simulink model "RA_Modes_Serial_HH"  (R2022b)
settings: Solver=FixedStepAuto  StartTime=0.0  StopTime=10.0  FixedStep=1e-3  RelTol=1e-3  EnableMultiTasking=on
undefined symbols (not defined in the file): A0, A1, D0, D1, D10, D11, D12, D13, D2, D3, D5, D6, D8, D9, PTA0, PTA1, PTA2, PTB2, PTB3, PTB9, PTC16, PTC17, PTC2, PTC4, PTD0, PTD1, PTD2, PTD3
libraries: etargetslib x22, frdmk64flib x20, dspstat3 x1
settings Model: ExtModeTrigDuration=5  Creator=haotianxue  LastModifiedBy=sarahalabdulrazzak
settings OptimizationCC: EnhancedBackFolding=on  PassReuseOutputArgsAs=Individual arguments  ZeroExternalMemoryAtStartup=off  ZeroInternalMemoryAtStartup=off  MaxStackSize=64  OptimizeBlockOrder=speed  DifferentSizesBufferReuse=on  OptimizationCustomize=off  EfficientTunableParamExpr=on
settings DebuggingCC: ParameterTunabilityLossMsg=error  UnconnectedInputMsg=warning  UnconnectedOutputMsg=warning  UnconnectedLineMsg=warning
settings HardwareCC: ProdBitPerPointer=32  ProdBitPerSizeT=32  ProdBitPerPtrDiffT=32  ProdLargestAtomicInteger=Long  ProdLargestAtomicFloat=Double  ProdWordSize=32  ProdHWDeviceType=ARM Compatible->ARM Cortex
settings ModelReferenceCC: EnableRefExpFcnMdlSchedulingChecks=on
settings SFSimCC: MATLABDynamicMemAlloc=off
settings RTWCC: Description=Embedded Coder  SystemTargetFile=ert.tlc  HardwareBoard=NXP FRDM-K64F  TLCOptions="-aInlineSetEventsForThisBaseRateFcn=TLC_FALSE -aSuppressMultiTaskScheduler=TLC_FALSE  -aRateBasedStepFcn=0"  TemplateMakefile=ert_default_tmf  Toolchain=GNU Tools for ARM Embedded Processors  DLArmComputeVersion=19.05
settings CodeAppCC: ForceParamTrailComments=on  IgnoreCustomStorageClasses=off  OperatorAnnotations=on  SimulinkDataObjDesc=on  SFDataObjDesc=on  InsertBlockDesc=on
settings ERTTargetCC: ExtModeTransport=4  ExtModeMexFile=sendToCommService

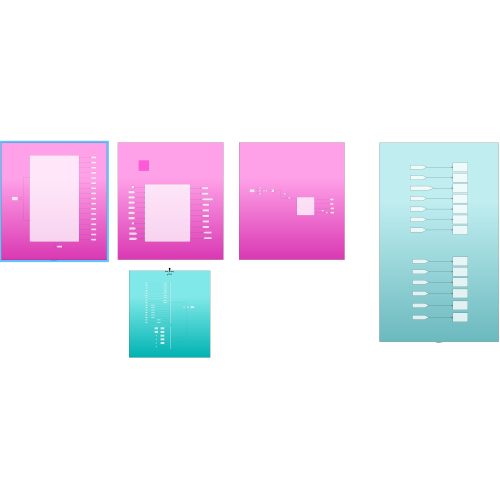
[thumbnail: Simulink's stored preview of the top-level diagram]
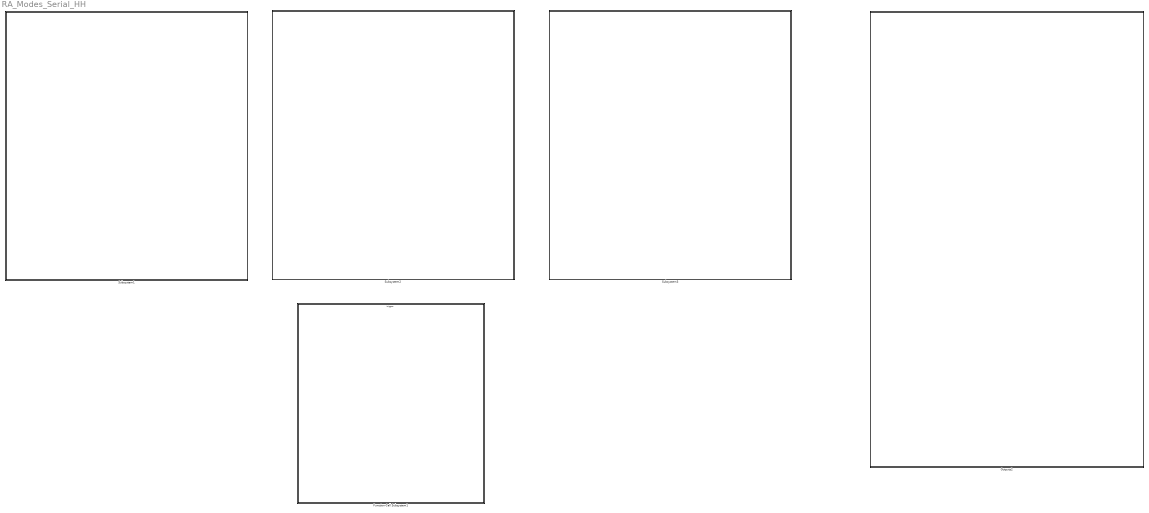
== system RA_Modes_Serial_HH ==
  Function-Call Subsystem1 : Subsystem  TreatAsAtomicUnit=on
  Outputs2 : Subsystem
  Subsystem1 : Subsystem
  Subsystem2 : Subsystem
  Subsystem3 : Subsystem

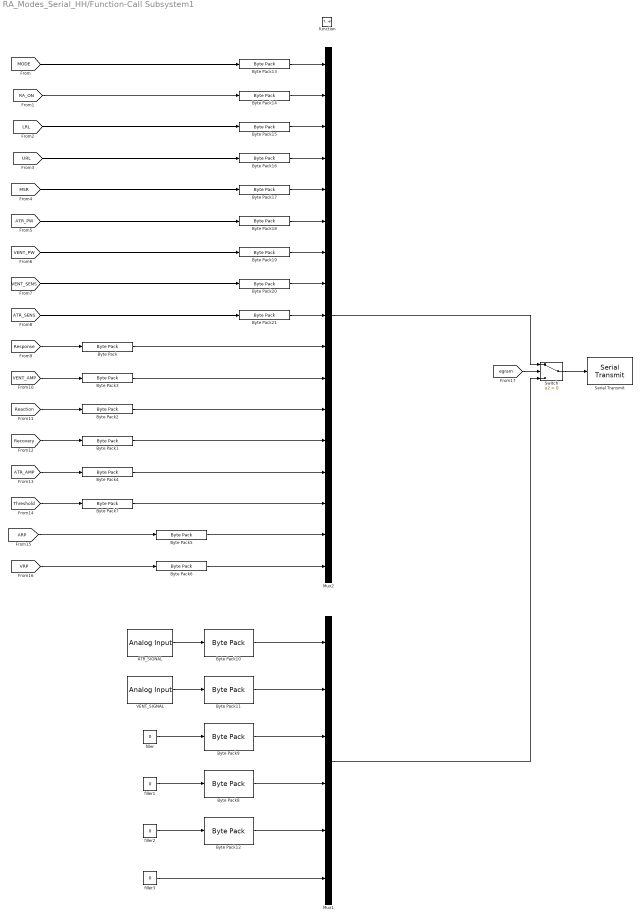
== system RA_Modes_Serial_HH/Function-Call Subsystem1 ==
  function : TriggerPort  TriggerType=function-call  IsSimulinkFunction=on  FunctionName=send_params  VariantControl=(inherit)
  ATR_SIGNAL : frdmk64flib/Analog Input  Whichpin=PTB2 (A0)  SampleTime=-1
  Byte Pack{,1..4,7,12} (7 alike) : etargetslib/Byte Pack  datatypes={'single'}  byteAlign=1
  Byte Pack{8..11} (4 alike) : etargetslib/Byte Pack  datatypes={'double'}  byteAlign=1
  Byte Pack{13..21} (9 alike) : etargetslib/Byte Pack  datatypes={'uint8'}  byteAlign=1
  Byte Pack5 : etargetslib/Byte Pack  datatypes={'uint16'}  byteAlign=1
  Byte Pack6 : etargetslib/Byte Pack  datatypes={'uint16'}  byteAlign=1
  Mux1 : Mux  Inputs=6
  Mux2 : Mux  Inputs=17
  Serial Transmit : frdmk64flib/Serial Transmit  SCIModule=0  Baudrate=uint32(9600)  Parity=None  StopBits=1  HardwareFlowControl=None  ByteOrder=LittleEndian  BlockingMode=on  OutputStatus=off
  Switch : Switch  Criteria=u2 > Threshold  SaturateOnIntegerOverflow=off  InputSameDT=off
  VENT_SIGNAL : frdmk64flib/Analog Input  Whichpin=PTB3 (A1)  SampleTime=-1
  filler : Constant  Value=0  OutDataTypeStr=double
  filler1 : Constant  Value=0  OutDataTypeStr=double
  filler2 : Constant  Value=0  OutDataTypeStr=single
  filler3 : Constant  Value=0  OutDataTypeStr=uint8
  wires:
  [VENT_SENS] -> Byte Pack20/1
  [ATR_SENS] -> Byte Pack21/1
  Byte Pack/1 -> Mux2/10
  Byte Pack1/1 -> Mux2/13
  Byte Pack2/1 -> Mux2/12
  Byte Pack3/1 -> Mux2/11
  Byte Pack4/1 -> Mux2/14
  Byte Pack5/1 -> Mux2/16
  Byte Pack6/1 -> Mux2/17
  [MODE] -> Byte Pack13/1
  [RA_ON] -> Byte Pack14/1
  [LRL] -> Byte Pack15/1
  [URL] -> Byte Pack16/1
  [MSR] -> Byte Pack17/1
  [ATR_PW] -> Byte Pack18/1
  [VENT_PW] -> Byte Pack19/1
  [Response] -> Byte Pack/1
  [VENT_AMP] -> Byte Pack3/1
  [Reaction] -> Byte Pack2/1
  [Recovery] -> Byte Pack1/1
  [ATR_AMP] -> Byte Pack4/1
  Byte Pack7/1 -> Mux2/15
  [Threshold] -> Byte Pack7/1
  [ARP] -> Byte Pack5/1
  [VRP] -> Byte Pack6/1
  Switch/1 -> Serial Transmit/1
  Mux2/1 -> Switch/1
  ATR_SIGNAL/1 -> Byte Pack10/1
  VENT_SIGNAL/1 -> Byte Pack11/1
  Mux1/1 -> Switch/3
  Byte Pack10/1 -> Mux1/1
  Byte Pack11/1 -> Mux1/2
  Byte Pack8/1 -> Mux1/4
  Byte Pack9/1 -> Mux1/3
  filler/1 -> Byte Pack9/1
  filler1/1 -> Byte Pack8/1
  Byte Pack12/1 -> Mux1/5
  filler2/1 -> Byte Pack12/1
  filler3/1 -> Mux1/6
  Byte Pack13/1 -> Mux2/1
  Byte Pack14/1 -> Mux2/2
  Byte Pack15/1 -> Mux2/3
  Byte Pack16/1 -> Mux2/4
  Byte Pack17/1 -> Mux2/5
  Byte Pack18/1 -> Mux2/6
  Byte Pack19/1 -> Mux2/7
  Byte Pack20/1 -> Mux2/8
  Byte Pack21/1 -> Mux2/9
  [egram] -> Switch/2

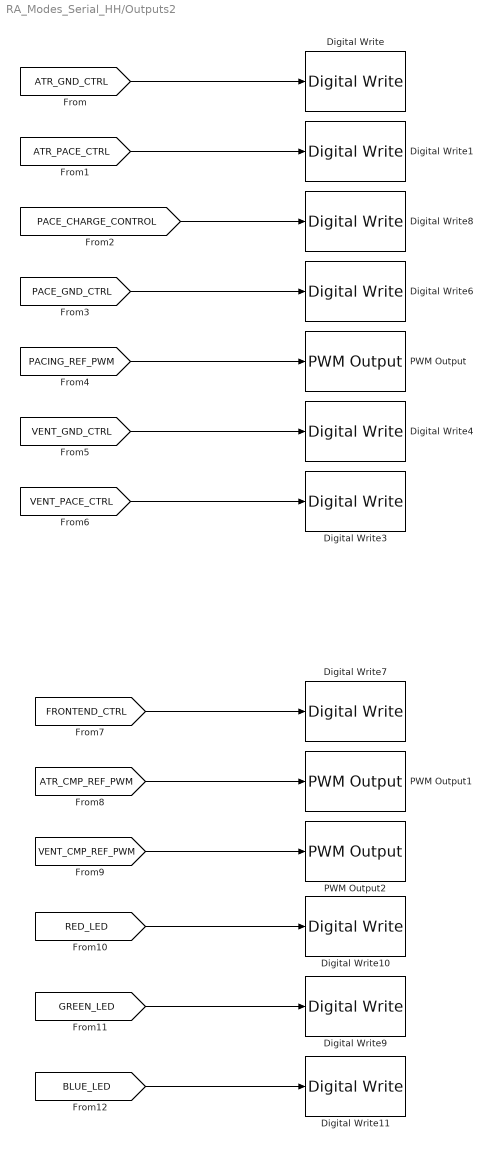
== system RA_Modes_Serial_HH/Outputs2 ==
  Digital Write : frdmk64flib/Digital Write  Whichpin=PTD2 (D11)
  Digital Write1 : frdmk64flib/Digital Write  Whichpin=PTA0 (D8)
  Digital Write10 : frdmk64flib/Digital Write  Whichpin=RED_LED
  Digital Write11 : frdmk64flib/Digital Write  Whichpin=BLUE_LED
  Digital Write3 : frdmk64flib/Digital Write  Whichpin=PTC4 (D9)
  Digital Write4 : frdmk64flib/Digital Write  Whichpin=PTD3 (D12)
  Digital Write6 : frdmk64flib/Digital Write  Whichpin=PTD0 (D10)
  Digital Write7 : frdmk64flib/Digital Write  Whichpin=PTD1 (D13)
  Digital Write8 : frdmk64flib/Digital Write  Whichpin=PTB9 (D2)
  Digital Write9 : frdmk64flib/Digital Write  Whichpin=GREEN_LED
  PWM Output : frdmk64flib/PWM Output  Whichpin=PTA2 (D5)  InitialFrequency=2000  InitialDutyCycle=0
  PWM Output1 : frdmk64flib/PWM Output  Whichpin=PTC2 (D6)  InitialFrequency=2000  InitialDutyCycle=0
  PWM Output2 : frdmk64flib/PWM Output  Whichpin=PTA1 (D3)  InitialFrequency=2000  InitialDutyCycle=0
  wires:
  [ATR_GND_CTRL] -> Digital Write/1
  [ATR_PACE_CTRL] -> Digital Write1/1
  [RED_LED] -> Digital Write10/1
  [GREEN_LED] -> Digital Write9/1
  [BLUE_LED] -> Digital Write11/1
  [PACE_GND_CTRL] -> Digital Write6/1
  [PACING_REF_PWM] -> PWM Output/1
  [VENT_GND_CTRL] -> Digital Write4/1
  [VENT_PACE_CTRL] -> Digital Write3/1
  [FRONTEND_CTRL] -> Digital Write7/1
  [ATR_CMP_REF_PWM] -> PWM Output1/1
  [VENT_CMP_REF_PWM] -> PWM Output2/1
  [PACE_CHARGE_CONTROL] -> Digital Write8/1

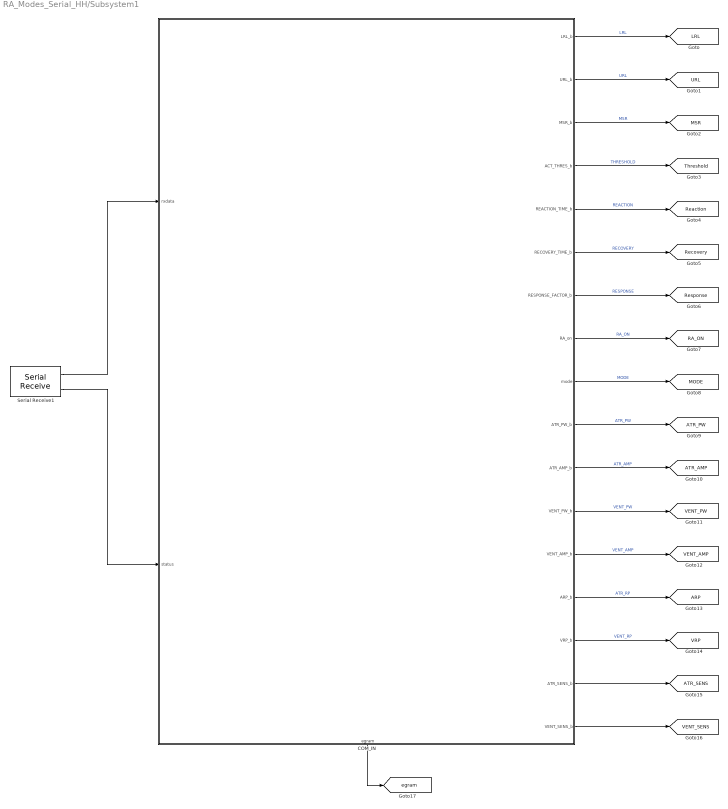
== system RA_Modes_Serial_HH/Subsystem1 ==
  COM_IN : Stateflow chart  TreatAsAtomicUnit=on
      settings: PortSchema="{\"entries\":[{\"content\":{\"sides\":[{\"content\":{\"connectorIds\":[\"In1\",\"In2\"]},\"type\":\"ConnectorPlacement.EquallySpacedRectSide\",\"uuid\":\"8214c444-1de1-4d31-bdd0-fdf28bd65edf\"},{\"content\":{\"connectorIds\":[\"Out1\",\"Out2\",\"Out3\",\"Out4\",\"Out5\",\"Out6\",\"Out7\",\"Out8\",\"Out9\",\"Out10\",\"Out11\",\"Out12\",\"Out13\",\"Out14\",\"Out15\",\"Out16\",\"Out17\"],\"side\":\"RIGHT\"},\"type\":\"ConnectorPlacement.EquallySpacedRectSide\",\"uuid\":\"fd4b820b-d988-4087-aa44-295b159a4f83\"},{\"content\":{\"connectorIds\":[],\"side\":\"TOP\"},\"type\":\"ConnectorPlacement.EquallySpacedRectSide\",\"uuid\":\"9cb3f67b-9bed-4d96-a295-eb351e913ea4\"},{\"content\":{\"connectorIds\":[\"Out18\"],\"side\":\"BOTTOM\"},\"type\":\"ConnectorPlacement.EquallySpacedRectSide\",\"uuid\":\"87181d9a-e9d0-4f8b-bc10-3b203b2fc102\"}]},\"type\":\"ConnectorPlacement.EquallySpacedConnector\",\"uuid\":\"39350b03-ea46-4b33-9d0b-af5e3b674f3a\"}],\"packageUris\":[\"http://schema.mathworks.com/mf0/Connector/R2020b\"],\"version\":\"1.0\"}"
  Serial Receive1 : frdmk64flib/Serial Receive  SCIModule=0  Baudrate=uint32(9600)  Parity=None  StopBits=1  HardwareFlowControl=None  ByteOrder=LittleEndian  DataType=uint8  DataLength=36  BlockingMode=off  OutputStatus=on  SampleTime=-1
  tag scope: ARP=global, ATR_AMP=global, ATR_PW=global, ATR_SENS=global, LRL=global, MODE=global, MSR=global, RA_ON=global, Reaction=global, Recovery=global, Response=global, Threshold=global, URL=global, VENT_AMP=global, VENT_PW=global, VENT_SENS=global, VRP=global, egram=global
  wires:
  Serial Receive1/2 -> COM_IN/2(status)
  Serial Receive1/1 -> COM_IN/1(rxdata)
  COM_IN/1(LRL_b) -> [LRL]  "LRL"
  COM_IN/2(URL_b) -> [URL]  "URL"
  COM_IN/3(MSR_b) -> [MSR]  "MSR"
  COM_IN/4(ACT_THRES_b) -> [Threshold]  "THRESHOLD"
  COM_IN/5(REACTION_TIME_b) -> [Reaction]  "REACTION"
  COM_IN/6(RECOVERY_TIME_b) -> [Recovery]  "RECOVERY"
  COM_IN/7(RESPONSE_FACTOR_b) -> [Response]  "RESPONSE"
  COM_IN/8(RA_on) -> [RA_ON]  "RA_ON"
  COM_IN/9(mode) -> [MODE]  "MODE"
  COM_IN/10(ATR_PW_b) -> [ATR_PW]  "ATR_PW"
  COM_IN/11(ATR_AMP_b) -> [ATR_AMP]  "ATR_AMP"
  COM_IN/12(VENT_PW_b) -> [VENT_PW]  "VENT_PW"
  COM_IN/13(VENT_AMP_b) -> [VENT_AMP]  "VENT_AMP"
  COM_IN/14(ARP_b) -> [ARP]  "ATR_RP"
  COM_IN/15(VRP_b) -> [VRP]  "VENT_RP"
  COM_IN/16(ATR_SENS_b) -> [ATR_SENS]
  COM_IN/17(VENT_SENS_b) -> [VENT_SENS]
  COM_IN/18(egram) -> [egram]

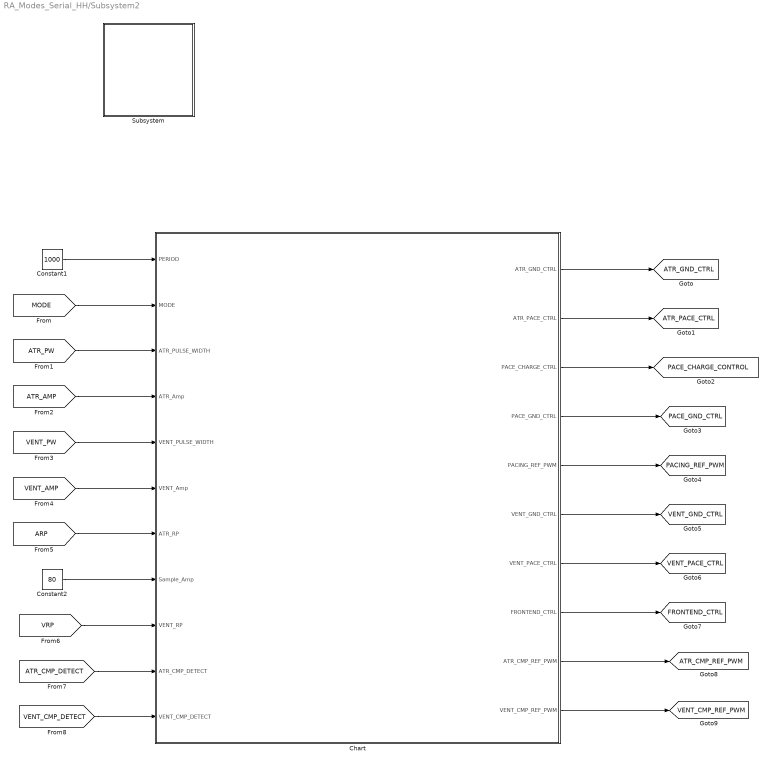
== system RA_Modes_Serial_HH/Subsystem2 ==
  Chart : Stateflow chart  TreatAsAtomicUnit=on
  Constant1 : Constant  Value=1000
  Constant2 : Constant  Value=80
  Subsystem : Subsystem
  tag scope: ATR_CMP_REF_PWM=global, ATR_GND_CTRL=global, ATR_PACE_CTRL=global, FRONTEND_CTRL=global, PACE_CHARGE_CONTROL=global, PACE_GND_CTRL=global, PACING_REF_PWM=global, VENT_CMP_REF_PWM=global, VENT_GND_CTRL=global, VENT_PACE_CTRL=global
  wires:
  Constant2/1 -> Chart/8(Sample_Amp)
  Constant1/1 -> Chart/1(PERIOD)
  [MODE] -> Chart/2(MODE)
  [ATR_PW] -> Chart/3(ATR_PULSE_WIDTH)
  [ATR_AMP] -> Chart/4(ATR_Amp)
  [VENT_PW] -> Chart/5(VENT_PULSE_WIDTH)
  [VENT_AMP] -> Chart/6(VENT_Amp)
  [ARP] -> Chart/7(ATR_RP)
  [VRP] -> Chart/9(VENT_RP)
  [ATR_CMP_DETECT] -> Chart/10(ATR_CMP_DETECT)
  [VENT_CMP_DETECT] -> Chart/11(VENT_CMP_DETECT)
  Chart/1(ATR_GND_CTRL) -> [ATR_GND_CTRL]
  Chart/2(ATR_PACE_CTRL) -> [ATR_PACE_CTRL]
  Chart/3(PACE_CHARGE_CTRL) -> [PACE_CHARGE_CONTROL]
  Chart/4(PACE_GND_CTRL) -> [PACE_GND_CTRL]
  Chart/5(PACING_REF_PWM) -> [PACING_REF_PWM]
  Chart/6(VENT_GND_CTRL) -> [VENT_GND_CTRL]
  Chart/7(VENT_PACE_CTRL) -> [VENT_PACE_CTRL]
  Chart/8(FRONTEND_CTRL) -> [FRONTEND_CTRL]
  Chart/9(ATR_CMP_REF_PWM) -> [ATR_CMP_REF_PWM]
  Chart/10(VENT_CMP_REF_PWM) -> [VENT_CMP_REF_PWM]

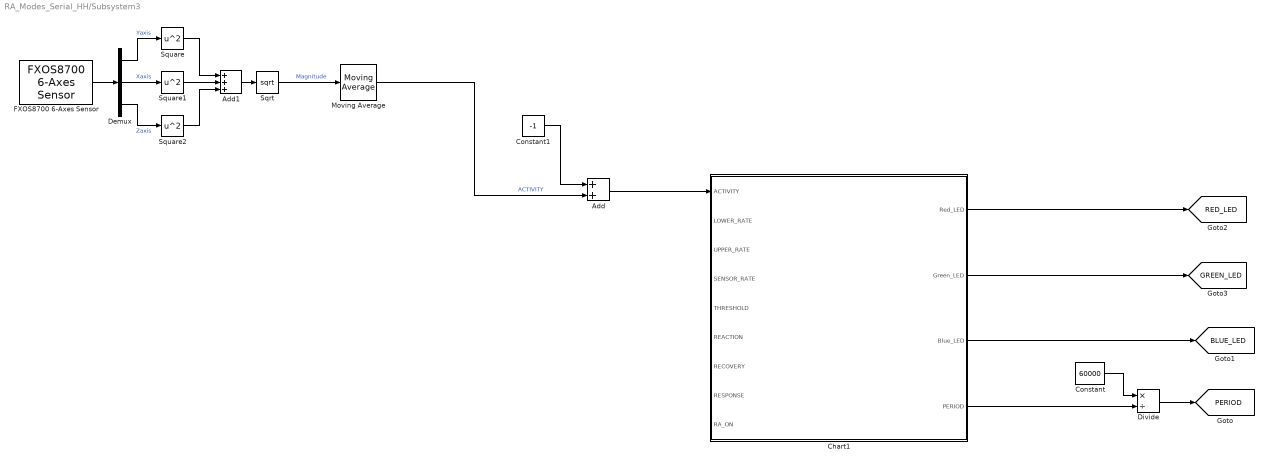
== system RA_Modes_Serial_HH/Subsystem3 ==
  Add : Sum
  Add1 : Sum  Inputs=+++
  Chart1 : Stateflow chart  TreatAsAtomicUnit=on
  Constant : Constant  Value=60000
  Constant1 : Constant  Value=-1
  Demux : Demux  Outputs=3
  Divide : Product  Inputs=*/
  FXOS8700 6-Axes Sensor : frdmk64flib/FXOS8700 6-Axes Sensor  Activesensor=Accelerometer only  ODR=800Hz  HybridODR=400Hz  Accelfullrange=-4g to +4g  SampleTime=-1
  Moving Average : dspstat3/Moving Average  Method=Exponential weighting  ForgettingFactorPort=off  SpecifyWindowLength=on  WindowLength=4  OverlapLength=3  AllowArbitraryInputLength=off  ForgettingFactor=0.999  SimulateUsing=Code generation
  Sqrt : Sqrt
  Square : Math  Operator=square
  Square1 : Math  Operator=square
  Square2 : Math  Operator=square
  tag scope: BLUE_LED=global, GREEN_LED=global, PERIOD=global, RED_LED=global
  wires:
  Add/1 -> Chart1/1(ACTIVITY)
  Square1/1 -> Add1/2
  Constant1/1 -> Add/1
  Constant/1 -> Divide/1
  Square/1 -> Add1/1
  Demux/1 -> Square/1  "Yaxis"
  Add1/1 -> Sqrt/1
  Moving Average/1 -> Add/2  "ACTIVITY"
  Square2/1 -> Add1/3
  Sqrt/1 -> Moving Average/1  "Magnitude"
  Demux/3 -> Square2/1  "Zaxis"
  Demux/2 -> Square1/1  "Xaxis"
  FXOS8700 6-Axes Sensor/1 -> Demux/1
  Chart1/4(PERIOD) -> Divide/2
  Divide/1 -> [PERIOD]
  Chart1/3(Blue_LED) -> [BLUE_LED]
  Chart1/2(Green_LED) -> [GREEN_LED]
  Chart1/1(Red_LED) -> [RED_LED]

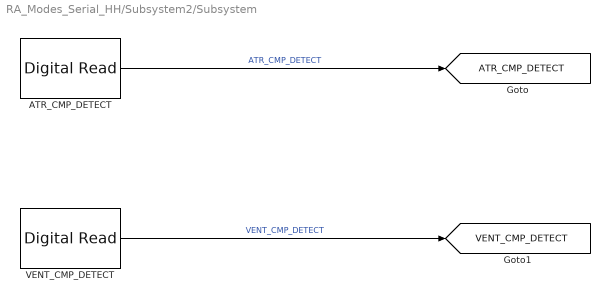
== system RA_Modes_Serial_HH/Subsystem2/Subsystem ==
  ATR_CMP_DETECT : frdmk64flib/Digital Read  Whichpin=PTC16 (D0)  SampleTime=-1
  VENT_CMP_DETECT : frdmk64flib/Digital Read  Whichpin=PTC17 (D1)  SampleTime=-1
  tag scope: ATR_CMP_DETECT=global, VENT_CMP_DETECT=global
  wires:
  VENT_CMP_DETECT/1 -> [VENT_CMP_DETECT]  "VENT_CMP_DETECT"
  ATR_CMP_DETECT/1 -> [ATR_CMP_DETECT]  "ATR_CMP_DETECT"

== stateflow chart RA_Modes_Serial_HH/Subsystem3/Chart1 ==
  state RECOVER_RATE
    %this is for if the RA is turned off while the
    %slowly shift activity (might not need)
    %if the period is above LRL, reduce by amount that will bring diff to 0 within recovery time
    Green_LED = true
    AVG_ACT = ACTIVITY
    if PERIOD > single(LOWER_RATE)
    PERIOD = PERIOD - (single(SENSOR_RATE)-single(LOWER_RATE))/(RECOVERY*60*1000)
    DELAY = (RECOVERY*60*1000)
    else
    PERIOD = single(LOWER_RATE)
    DELAY = single(0)
    end
  state RA_OFF
    %set the period to LRL
    %read current activity
    %and assign to var.
    entry:
    PERIOD = single(LOWER_RATE)
    AVG_ACT = ACTIVITY
    TH = single(THRESHOLD)
    if PERIOD >= 60
    Red_LED = true
    elseif PERIOD < 60
    Red_LED = false
    end
  state SET_TARGET
    %set the target rate and make sure it falls within the bounds
    Green_LED = false
    Red_LED = true
    TARGET_RATE = RESPONSE*((single(SENSOR_RATE) - single(LOWER_RATE))/10)*ACTIVITY + single(LOWER_RATE)
    %TARGET_RATE = 120
    if TARGET_RATE > single(SENSOR_RATE)
    TARGET_RATE = single(SENSOR_RATE)
    elseif TARGET_RATE < single(LOWER_RATE)
    TARGET_RATE = single(LOWER_RATE)
    end
  state RA_ON
    entry:
    Blue_LED = false
    Green_LED = false
    Red_LED = false
  state RECOVER_REACT
    %slowly shift activity (might not need)
    %if Period is above target, decrease using recovery
    %if below target, increase using reaction
    Blue_LED = true
    AVG_ACT = ACTIVITY
    if PERIOD > TARGET_RATE
    PERIOD = PERIOD - (single(SENSOR_RATE)-single(LOWER_RATE))/(RECOVERY*60*1000)
    DELAY = (RECOVERY*60*1000)
    elseif PERIOD < TARGET_RATE
    PERIOD = PERIOD + (single(SENSOR_RATE)-single(LOWER_RATE))/(REACTION*1000)
    DELAY = (REACTION*1000)
    end
  RECOVER_RATE -> SET_TARGET [order 1] : [n >= DELAY && AVG_ACT >= TH]
  RECOVER_RATE -> RECOVER_RATE [order 2] : after(1,msec){n = n+1}
  RECOVER_RATE -> RA_OFF [order 3] : [RA_ON == FALSE && n >= DELAY]
  RA_ON -> RECOVER_RATE [order 1] : [AVG_ACT < TH]{n=0}
  (default) -> RA_OFF
  RA_ON -> SET_TARGET [order 2] : [AVG_ACT >= TH]
  RA_OFF -> RA_ON : [RA_ON == TRUE]{TARGET_RATE=PERIOD}
  RECOVER_REACT -> RA_ON [order 1] : [n >= DELAY]
  SET_TARGET -> RECOVER_REACT : {n=0, AVG_ACT = ACTIVITY}
  RECOVER_REACT -> RECOVER_REACT [order 2] : after(1,msec){n = n+1}
  data: ACTIVITY input; LOWER_RATE input; UPPER_RATE input; SENSOR_RATE input; THRESHOLD input; REACTION input; RECOVERY input; RESPONSE input; RA_ON input; TRUE local =1; FALSE local =0; TARGET_RATE local; DELAY local; n local; Red_LED output; Green_LED output; Blue_LED output; PERIOD output; TH local; AVG_ACT local

== stateflow chart RA_Modes_Serial_HH/Subsystem1/COM_IN ==
  state SET_PARAM
    entry:
    %red_en = rxdata(3);
    %green_en =  rxdata(4);
    %blue_en = rxdata(5);
    %off_time = typecast(rxdata(6:9), 'single');
    %switch_time = typecast(rxdata(10:11), 'uint16');
    egram = 1;
    mode = rxdata(3);
    RA_on = rxdata(4);
    LRL_b = rxdata(5)
    URL_b = rxdata(6);
    MSR_b = rxdata(7);
    ATR_PW_b = rxdata(8);
    VENT_PW_b = rxdata(9);
    VENT_SENS_b = rxdata(10);
    ATR_SENS_b = rxdata(11);
    RESPONSE_FACTOR_b = typecast(rxdata(12:15), 'single');
    VENT_AMP_b = typecast(rxdata(16:19), 'single');
    REACTION_TIME_b = typecast(rxdata(20:23), 'single');
    RECOVERY_TIME_b = typecast(rxdata(24:27), 'single');
    ATR_AMP_b = typecast(rxdata(28:31), 'single')
    ACT_THRES_b = typecast(rxdata(32:35), 'single');
    ARP_b = typecast(rxdata(36:37), 'uint16');
    VRP_b = typecast(rxdata(38:39), 'uint16');
  state INITIAL
    entry:
    %red_en = 1;
    %green_en = 1;
    %blue_en = 1;
    %off_time = 0.5;
    %switch_time = 200;
    URL_b = uint8(120);
    LRL_b = uint8(60);
    MSR_b = uint8(120);
    mode = uint8(1);
    RA_on = uint8(0);
    ATR_PW_b = uint8(5);
    ATR_AMP_b = single(3.75);
    VENT_PW_b = uint8(5);
    VENT_AMP_b = single(3.75);
    ARP_b = uint16(250);
    VRP_b = uint16(350);
    VENT_SENS_b = uint8(2);
    ATR_SENS_b = uint8(1);
    REACTION_TIME_b = single(30.0);
    RECOVERY_TIME_b = single(5.0);
    RESPONSE_FACTOR_b = single(8.0);
    ACT_THRES_b = single(1.2);
  state SEND_EGRAM
    entry:
    egram = 0
    send_params()
  state STANDBY
    entry:
    egram = 1
  state ECHO_PARAM
    entry:
    send_params();
  (default) -> INITIAL
  SET_PARAM -> STANDBY
  (junction 15) -> SET_PARAM [order 1] : [rxdata(2)==hex2dec('55')]
  (junction 14) -> STANDBY [order 2]
  INITIAL -> STANDBY
  STANDBY -> (junction 14) : [status==0]
  (junction 14) -> (junction 15) [order 1] : [rxdata(1)==hex2dec('16')]
  (junction 15) -> SEND_EGRAM [order 3] : [rxdata(2)==hex2dec('47')]
  SEND_EGRAM -> STANDBY
  (junction 15) -> ECHO_PARAM [order 2] : [rxdata(2)==hex2dec('22')]
  ECHO_PARAM -> STANDBY
  data: LRL_b output uint8; URL_b output uint8; MSR_b output uint8; rxdata input uint8; status input uint8; ACT_THRES_b output single; REACTION_TIME_b output single; RECOVERY_TIME_b output single; RESPONSE_FACTOR_b output single; RA_on output uint8; mode output uint8; ATR_PW_b output uint8; ATR_AMP_b output single; VENT_PW_b output uint8; VENT_AMP_b output single; ARP_b output uint16; VRP_b output uint16; ATR_SENS_b output uint8; VENT_SENS_b output uint8; egram output

== stateflow chart RA_Modes_Serial_HH/Subsystem2/Chart ==
  state Identify_Mode_Path1
    entry:
    % MODE = 1 (AOO)
    % MODE = 2 (AAI)
    % MODE = 3 (VOO)
    % MODE = 4 (VVI)
    %
    %pacemaker disconnected
    %stop sensing
    PACE_CHARGE_CTRL = LOW
    VENT_PACE_CTRL = LOW
    ATR_PACE_CTRL = LOW
    PACE_GND_CTRL = LOW
    ATR_GND_CTRL = LOW
    VENT_GND_CTRL = LOW
    FRONTEND_CTRL = LOW
  state AOO1
    entry:
    %Charge primary capcitor C22
    ATR_PACE_CTRL=LOW
    PACING_REF_PWM = 20*ATR_Amp
    PACE_CHARGE_CTRL = HIGH
    %Discharge block capacitor C21
    PACE_GND_CTRL = HIGH
    ATR_GND_CTRL = HIGH
    %use LED  to verify state
  state AOO_ATR_PULSE1
    entry:
    %Discharge C22 primary capacitor
    %Charge C21 block capacitor
    PACE_CHARGE_CTRL = LOW
    PACE_GND_CTRL = HIGH
    ATR_PACE_CTRL = HIGH
    ATR_GND_CTRL = LOW
    PACING_REF_PWM = 20*ATR_Amp
    %use LED  to verify state
  state AAI_ATR_PULSE1
    entry:
    %sensing OFF
    FRONTEND_CTRL = LOW
    %Discharge C22 primary capacitor
    %Charge C21 block capacitor
    PACE_CHARGE_CTRL = LOW
    PACE_GND_CTRL = HIGH
    ATR_PACE_CTRL = HIGH
    ATR_GND_CTRL = LOW
    PACING_REF_PWM = 20*ATR_Amp
    %use LED  to verify state
  state AAI1
    entry:
    %sensing ON
    FRONTEND_CTRL = HIGH
    %Charge primary capcitor C22
    ATR_PACE_CTRL=LOW
    PACING_REF_PWM = 20*ATR_Amp
    PACE_CHARGE_CTRL = HIGH
    %Discharge block capacitor C21
    PACE_GND_CTRL = HIGH
    ATR_GND_CTRL = HIGH
    ATR_CMP_REF_PWM = Sample_Amp
    %use LED  to verify state
  state VOO1
    entry:
    %Charge primary capcitor C22
    VENT_PACE_CTRL=LOW
    PACING_REF_PWM = 20*VENT_Amp
    PACE_CHARGE_CTRL = HIGH
    %Discharge block capacitor C21
    PACE_GND_CTRL = HIGH
    VENT_GND_CTRL = HIGH
    %use LED  to verify state
  state VOO_VENT_PULSE1
    entry:
    %Discharge C22 primary capacitor
    %Charge C21 block capacitor
    PACE_CHARGE_CTRL = LOW
    PACE_GND_CTRL = HIGH
    VENT_GND_CTRL = LOW
    VENT_PACE_CTRL  = HIGH
    PACING_REF_PWM = 20*VENT_Amp
    %use LED  to verify state
  state VVI1
    entry:
    %sensing ON
    FRONTEND_CTRL = HIGH
    %Charge primary capcitor C22
    VENT_PACE_CTRL= LOW
    PACING_REF_PWM = 20*VENT_Amp
    PACE_CHARGE_CTRL = HIGH
    %Discharge block capacitor C21
    PACE_GND_CTRL = HIGH
    VENT_PACE_CTRL = LOW
    VENT_GND_CTRL = HIGH
    VENT_CMP_REF_PWM = Sample_Amp
    %use LED  to verify state
  state VVI_VENT_PULSE1
    %sensing OFF
    FRONTEND_CTRL = LOW
    %Discharge C22 primary capacitor
    %Charge C21 block capacitor
    PACE_CHARGE_CTRL = LOW
    PACE_GND_CTRL = HIGH
    VENT_GND_CTRL = LOW
    VENT_PACE_CTRL  = HIGH
    PACING_REF_PWM = 20*VENT_Amp
    %use LED  to verify state
  (default) -> Identify_Mode_Path1
  AOO1 -> AOO_ATR_PULSE1 [order 1] : after(PERIOD - ATR_PULSE_WIDTH,msec)
  Identify_Mode_Path1 -> AOO1 [order 1] : [MODE == 1]
  AOO_ATR_PULSE1 -> AOO1 : after(ATR_PULSE_WIDTH,msec)
  AOO1 -> Identify_Mode_Path1 [order 2] : [MODE ~= 1]
  AAI_ATR_PULSE1 -> AAI1 : after(ATR_PULSE_WIDTH,msec)
  Identify_Mode_Path1 -> AAI1 [order 2] : [MODE == 2]
  AAI1 -> (junction 113) [order 1]
  (junction 113) -> AAI_ATR_PULSE1 [order 1] : after(PERIOD - ATR_PULSE_WIDTH,msec)[ATR_CMP_DETECT == LOW]
  (junction 113) -> AAI1 [order 2] : after(ATR_RP, msec)[ATR_CMP_DETECT == HIGH]
  AAI1 -> Identify_Mode_Path1 [order 2] : [MODE ~= 2]
  VOO1 -> VOO_VENT_PULSE1 [order 1] : after(PERIOD - VENT_PULSE_WIDTH,msec)
  Identify_Mode_Path1 -> VOO1 [order 3] : [MODE == 3]
  VOO_VENT_PULSE1 -> VOO1 : after(VENT_PULSE_WIDTH,msec)
  VOO1 -> Identify_Mode_Path1 [order 2] : [MODE ~= 3]
  VVI_VENT_PULSE1 -> VVI1 : after(VENT_PULSE_WIDTH,msec)
  Identify_Mode_Path1 -> VVI1 [order 4] : [MODE == 4]
  VVI1 -> (junction 119) [order 1]
  (junction 119) -> VVI_VENT_PULSE1 [order 1] : after(PERIOD - VENT_PULSE_WIDTH,msec)[VENT_CMP_DETECT == LOW]
  (junction 119) -> VVI1 [order 2] : after(VENT_RP, msec)[VENT_CMP_DETECT == HIGH]
  VVI1 -> Identify_Mode_Path1 [order 2] : [MODE ~= 4]
  data: PERIOD input; MODE input; ATR_PULSE_WIDTH input; ATR_Amp input; VENT_PULSE_WIDTH input; VENT_Amp input; ATR_RP input; Sample_Amp input; VENT_RP input; ATR_CMP_DETECT input; VENT_CMP_DETECT input; HIGH local =1; LOW local =0; ATR_GND_CTRL output; ATR_PACE_CTRL output; PACE_CHARGE_CTRL output; PACE_GND_CTRL output; PACING_REF_PWM output; VENT_GND_CTRL output; VENT_PACE_CTRL output; FRONTEND_CTRL output; ATR_CMP_REF_PWM output; VENT_CMP_REF_PWM output
